simulink model "PIcomper"  (R2022b)
settings: Solver=FixedStepAuto  StartTime=0  StopTime=0.2  FixedStep=Ts  MaxStep=1e-5  RelTol=1e-5  EnableMultiTasking=on
InitFcn:
  | %% 原参数
  | Rs = 0.0135;      % 电阻
  | Ld = 5.45e-5;     % 电感
  | Ls = Ld;
  | Psi_f = 0.000639286;
  | 
  | %% 新参数
  | Rs = 0.44;
  | Ld = 0.2e-3;
  | Lq = Ld;
  | Ls = Ld;
  | Psi_f = 0.0112;
  | 
  | %% 公共参数
  | Ts = 1e-6;        % 采样时间
  | theta0 = 1.5;
  | F = 0;
  | P = 7;    % 磁极对数
  | np = P;
  | J = 1.05e-5;
  | Ud = 180; % 直流侧逆变电压。
undefined symbols (not defined in the file or in its folder): DiscIntNeverNeededParam
libraries: spsControlledVoltageSourceLib x6, spsMosfetLib x6, simulink x6, spsSeriesRLCBranchLib x3, spsCurrentMeasurementLib x3, spsVoltageMeasurementLib x3, spsDCVoltageSourceLib x1, spspowerguiLib x1, slpidlib x1, mcbcontrolslib x1
settings Model: Creator=hengst  LastModifiedBy=Administrator
settings SolverCC: AlgebraicLoopSolver=TrustRegion  AutoInsertRateTranBlk=on
settings DataIOCC: ReturnWorkspaceOutputs=off
settings OptimizationCC: LifeSpan=inf
settings DebuggingCC: UnconnectedInputMsg=warning  UnconnectedOutputMsg=warning  UnconnectedLineMsg=warning  SFUnexpectedBacktrackingDiag=warning  SFNoUnconditionalDefaultTransitionDiag=warning  ArithmeticOperatorsInVariantConditions=warning
settings ModelReferenceCC: EnableRefExpFcnMdlSchedulingChecks=on
settings SFSimCC: SimUseLocalCustomCode=off  CustomCodeUndefinedFunction=UseInterfaceOnly
settings RTWCC: RTWUseLocalCustomCode=off
settings CodeAppCC: StateflowObjectComments=on
settings GRTTargetCC: TargetLangStandard=C89/C90 (ANSI)
settings ConfigComp: CovMetricSettings=dw  CovSaveCumulativeToWorkspaceVar=on  CovSaveSingleToWorkspaceVar=on  CovExternalEMLEnable=off
settings SimscapeCC: SimscapeNormalizeSystem=off  SimscapeLogType=local

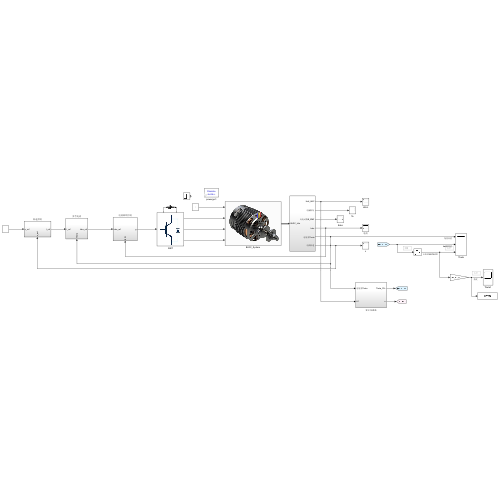
[thumbnail: Simulink's stored preview of the top-level diagram]
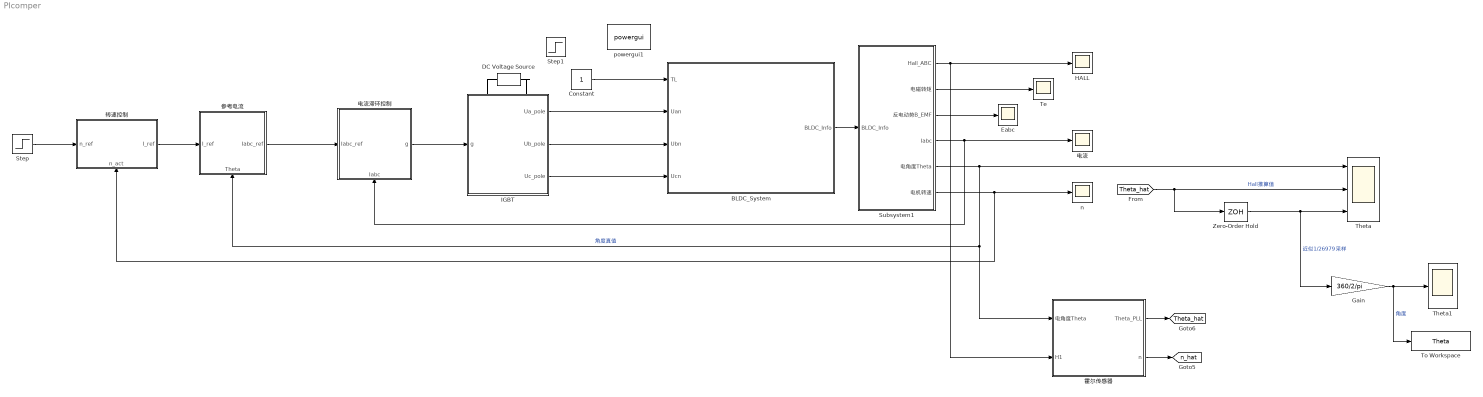
== system PIcomper ==
  BLDC_System : Subsystem
      mask Display: image('$imagefile');
  Constant : Constant
  DC Voltage Source : spsDCVoltageSourceLib/DC Voltage Source  Amplitude=Ud  Measurements=None
  Eabc : Scope
  Gain : Gain  Gain=360/2/pi
  HALL : Scope
  IGBT : Subsystem
      settings: PortSchema="{\"entries\":[{\"content\":{\"sides\":[{\"content\":{\"connectorIds\":[\"In1\"]},\"type\":\"ConnectorPlacement.EquallySpacedRectSide\",\"uuid\":\"41b52271-ff12-456f-8c0a-72ec256cd55e\"},{\"content\":{\"connectorIds\":[\"Out1\",\"Out2\",\"Out3\"],\"side\":\"RIGHT\"},\"type\":\"ConnectorPlacement.EquallySpacedRectSide\",\"uuid\":\"a3d71e7d-2158-4df1-810d-2282058bfce1\"},{\"content\":{\"connectorIds\":[\"LConn1\",\"LConn2\"],\"side\":\"TOP\"},\"type\":\"ConnectorPlacement.EquallySpacedRectSide\",\"uuid\":\"c64f7271-b3fd-4b5a-a4a2-aff74259f2ea\"}]},\"type\":\"ConnectorPlacement.EquallySpacedConnector\",\"uuid\":\"dfb04f65-d2fa-4b5c-99a8-719731ad9d2d\"}],\"packageUris\":[\"http://schema.mathworks.com/mf0/Connector/R2020b\"],\"version\":\"1.0\"}"
      mask Display: image('$imagefile'); % 使用工具条上的 "编辑图像" 进行更改。
  Step : Step  Time=0.1  Before=4000  After=2000
  Step1 : Step  Time=0.1
  Subsystem1 : Subsystem
  Te : Scope
  Theta : Scope  NumInputPorts=3
  Theta1 : Scope
  To Workspace : ToWorkspace  VariableName=Theta  SampleTime=-1
      settings: Save2DSignal=2-D array (concatenate along first dimension)
  Zero-Order Hold : ZeroOrderHold  SampleTime=3e-5
  n : Scope
  powergui1 : spspowerguiLib/powergui  Priority=1  SimulationMode=Discrete  SampleTime=Ts  frequency=60  Iterations=50  frequencyindice=0  Pbase=100e6  ErrMax=1e-4  UnitsV=kV  UnitsW=MW  buscounter=0  FunctionMessages=off  echomessages=off  EnableUseOfTLC=off  CurrentSourceSwitches=off  DisableSnubberDevices=off  DisableRonSwitches=off  DisableVfSwitches=off  DisplayEquations=off  AutomaticDiscreteSolvers=off  SolverType=Tustin/Backward Euler (TBE)  Interpol=off  ExternalGateDelay=off  methode=off  Ts=10  x0status=blocks  SPID=off  SwTol=0  HookPort=off  NonlinearTolerance=0  nMaxIteration=15  ContinueOnMaxIteration=off  RestoreLinks=warning  ResistiveCurrentMeasurement=off  Frange=[0:2:500]  Ylog=off  Xlog=on  ShowGrid=off  save=off  variable=ZData  structure=0  ZoomFFT=off  StartTime=0.0  cycles=1  DisplayStyle=1  fundamental=60  FreqAxis=off  MaxFrequency=1000  frequencyindicesteady=1  RmsSteady=1  display=off
  参考电流 : Subsystem
      settings: PortSchema="{\"entries\":[{\"content\":{\"sides\":[{\"content\":{\"connectorIds\":[\"In1\"]},\"type\":\"ConnectorPlacement.EquallySpacedRectSide\",\"uuid\":\"41f220d8-6130-485c-9e7a-1b6f64f24949\"},{\"content\":{\"connectorIds\":[\"Out1\"],\"side\":\"RIGHT\"},\"type\":\"ConnectorPlacement.EquallySpacedRectSide\",\"uuid\":\"42567a46-54e2-4998-94b6-634996524ad2\"},{\"content\":{\"side\":\"TOP\"},\"type\":\"ConnectorPlacement.EquallySpacedRectSide\",\"uuid\":\"fc447078-e630-4c42-83ce-d62d9e71be1e\"},{\"content\":{\"connectorIds\":[\"In2\"],\"side\":\"BOTTOM\"},\"type\":\"ConnectorPlacement.EquallySpacedRectSide\",\"uuid\":\"ba6e3960-44ca-42f2-94af-32e971d19e9e\"}]},\"type\":\"ConnectorPlacement.EquallySpacedConnector\",\"uuid\":\"b51f524c-61b9-4403-9c61-bea0d47ef62b\"}],\"packageUris\":[\"http://schema.mathworks.com/mf0/Connector/R2020b\"],\"version\":\"1.0\"}"
  电流 : Scope
  电流滞环控制 : Subsystem
      settings: PortSchema="{\"entries\":[{\"content\":{\"sides\":[{\"content\":{\"connectorIds\":[\"In1\"]},\"type\":\"ConnectorPlacement.EquallySpacedRectSide\",\"uuid\":\"41f220d8-6130-485c-9e7a-1b6f64f24949\"},{\"content\":{\"connectorIds\":[\"Out1\"],\"side\":\"RIGHT\"},\"type\":\"ConnectorPlacement.EquallySpacedRectSide\",\"uuid\":\"42567a46-54e2-4998-94b6-634996524ad2\"},{\"content\":{\"side\":\"TOP\"},\"type\":\"ConnectorPlacement.EquallySpacedRectSide\",\"uuid\":\"fc447078-e630-4c42-83ce-d62d9e71be1e\"},{\"content\":{\"connectorIds\":[\"In2\"],\"side\":\"BOTTOM\"},\"type\":\"ConnectorPlacement.EquallySpacedRectSide\",\"uuid\":\"84779085-48c1-4a07-a7e4-235775ba11f2\"}]},\"type\":\"ConnectorPlacement.EquallySpacedConnector\",\"uuid\":\"b51f524c-61b9-4403-9c61-bea0d47ef62b\"}],\"packageUris\":[\"http://schema.mathworks.com/mf0/Connector/R2020b\"],\"version\":\"1.0\"}"
  转速控制 : Subsystem
      settings: PortSchema="{\"entries\":[{\"content\":{\"sides\":[{\"content\":{\"connectorIds\":[\"In1\"]},\"type\":\"ConnectorPlacement.EquallySpacedRectSide\",\"uuid\":\"41f220d8-6130-485c-9e7a-1b6f64f24949\"},{\"content\":{\"connectorIds\":[\"Out1\"],\"side\":\"RIGHT\"},\"type\":\"ConnectorPlacement.EquallySpacedRectSide\",\"uuid\":\"42567a46-54e2-4998-94b6-634996524ad2\"},{\"content\":{\"side\":\"TOP\"},\"type\":\"ConnectorPlacement.EquallySpacedRectSide\",\"uuid\":\"fc447078-e630-4c42-83ce-d62d9e71be1e\"},{\"content\":{\"connectorIds\":[\"In2\"],\"side\":\"BOTTOM\"},\"type\":\"ConnectorPlacement.EquallySpacedRectSide\",\"uuid\":\"1fc4d12d-9707-4f98-a812-9cfaae9f9679\"}]},\"type\":\"ConnectorPlacement.EquallySpacedConnector\",\"uuid\":\"b51f524c-61b9-4403-9c61-bea0d47ef62b\"}],\"packageUris\":[\"http://schema.mathworks.com/mf0/Connector/R2020b\"],\"version\":\"1.0\"}"
  霍尔传感器 : Subsystem
  tag scope: Theta_hat=global, n_hat=global
  wires:
  参考电流/1(Iabc_ref) -> 电流滞环控制/1(Iabc_ref)
  电流滞环控制/1(g) -> IGBT/1(g)
  Subsystem1/6(电机转速) -> n/1, 转速控制/2(n_act)
  转速控制/1(I_ref) -> 参考电流/1(I_ref)
  Subsystem1/1(Hall_ABC) -> 霍尔传感器/2(H1), HALL/1
  BLDC_System/1(BLDC_Info) -> Subsystem1/1(BLDC_Info)
  Subsystem1/2(电磁转矩) -> Te/1
  Subsystem1/5(电角度Theta) -> Theta/1, 霍尔传感器/1(电角度Theta), 参考电流/2(Theta)  "角度真值"
  Subsystem1/4(Iabc) -> 电流/1, 电流滞环控制/2(Iabc)
  IGBT/1(Ua_pole) -> BLDC_System/2(Uan)
  IGBT/2(Ub_pole) -> BLDC_System/3(Ubn)
  IGBT/3(Uc_pole) -> BLDC_System/4(Ucn)
  Subsystem1/3(反电动势B_EMF) -> Eabc/1
  霍尔传感器/2(n) -> [n_hat]
  霍尔传感器/1(Theta_PLL) -> [Theta_hat]
  [Theta_hat] -> Zero-Order Hold/1, Theta/2  "Hall推算值"
  Zero-Order Hold/1 -> Gain/1, Theta/3  "近似1/26979采样"
  Gain/1 -> To Workspace/1, Theta1/1  "角度"
  Constant/1 -> BLDC_System/1(TL)
  Step/1 -> 转速控制/1(n_ref)
  connections:
  DC Voltage Source/RConn1 -- IGBT/LConn1
  DC Voltage Source/LConn1 -- IGBT/LConn2

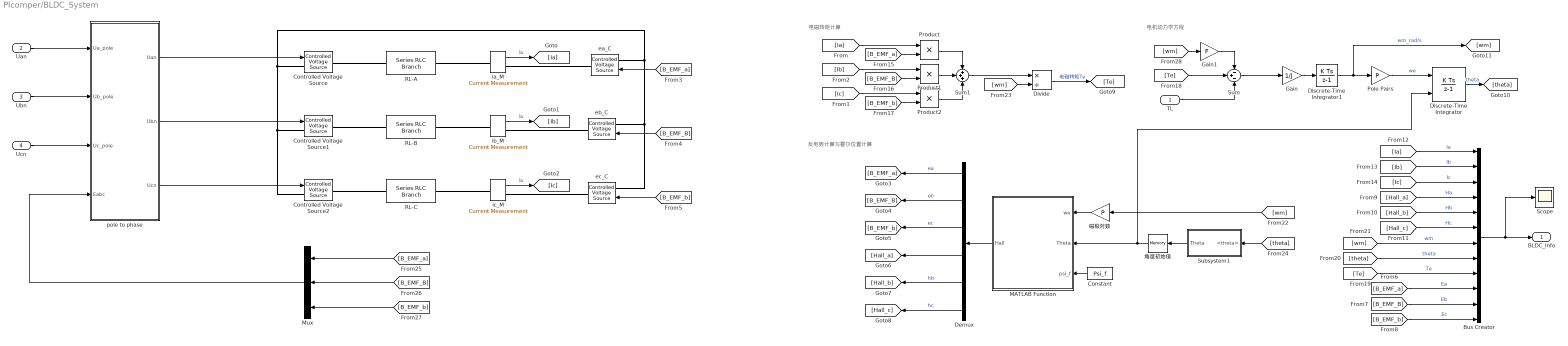
== system PIcomper/BLDC_System ==
  note: 反电势计算与霍尔位置计算
  note: 电磁转矩计算
  note: 电机动力学方程
  TL : Inport
  Uan : Inport  Port=2
  Ubn : Inport  Port=3
  Ucn : Inport  Port=4
  Bus Creator : BusCreator  Inputs=12
  Constant : Constant  Value=Psi_f
  Controlled Voltage Source : spsControlledVoltageSourceLib/Controlled Voltage Source  Initialize=on  Source_Type=AC  Amplitude=0  Phase=0  Frequency=0  Measurements=None
  Controlled Voltage Source1 : spsControlledVoltageSourceLib/Controlled Voltage Source  Initialize=on  Source_Type=AC  Amplitude=0  Phase=0  Frequency=0  Measurements=None
  Controlled Voltage Source2 : spsControlledVoltageSourceLib/Controlled Voltage Source  Initialize=on  Source_Type=AC  Amplitude=0  Phase=0  Frequency=0  Measurements=None
  Demux : Demux  Outputs=6
  Discrete-Time Integrator : DiscreteIntegrator  InitialConditionSource=external  SampleTime=-1  ICPrevOutput=DiscIntNeverNeededParam  ICPrevScaledInput=DiscIntNeverNeededParam
  Discrete-Time Integrator1 : DiscreteIntegrator  InitialCondition=1e-5  SampleTime=-1  ICPrevOutput=DiscIntNeverNeededParam  ICPrevScaledInput=DiscIntNeverNeededParam
  Divide : Product  Inputs=*/
  Gain : Gain  Gain=1/J
  Gain1 : Gain  Gain=F
  MATLAB Function : MATLAB Function  TreatAsAtomicUnit=on
  Mux : Mux  Inputs=3
  Pole Pairs : Gain  Gain=P
  Product : Product
  Product1 : Product
  Product2 : Product
  RL-A : spsSeriesRLCBranchLib/Series RLC Branch  LConnTagsString=__new0  RConnTagsString=__new0  BranchType=RL  Resistance=Rs  Inductance=Ls  SetiL0=off  InitialCurrent=0  Capacitance=1e-6  Setx0=off  InitialVoltage=0  Measurements=Branch voltage and current
  RL-B : spsSeriesRLCBranchLib/Series RLC Branch  LConnTagsString=__new0  RConnTagsString=__new0  BranchType=RL  Resistance=Rs  Inductance=Ls  SetiL0=off  InitialCurrent=0  Capacitance=1e-6  Setx0=off  InitialVoltage=0  Measurements=Branch voltage and current
  RL-C : spsSeriesRLCBranchLib/Series RLC Branch  LConnTagsString=__new0  RConnTagsString=__new0  BranchType=RL  Resistance=Rs  Inductance=Ls  SetiL0=off  InitialCurrent=0  Capacitance=1e-6  Setx0=off  InitialVoltage=0  Measurements=Branch voltage and current
  Scope : Scope
  Subsystem1 : Subsystem
  Sum : Sum  Inputs=-+-
  Sum1 : Sum  Inputs=+++
  ea_C : spsControlledVoltageSourceLib/Controlled Voltage Source  Initialize=on  Source_Type=AC  Amplitude=0  Phase=0  Frequency=0  Measurements=None
  eb_C : spsControlledVoltageSourceLib/Controlled Voltage Source  Initialize=on  Source_Type=AC  Amplitude=0  Phase=0  Frequency=0  Measurements=None
  ec_C : spsControlledVoltageSourceLib/Controlled Voltage Source  Initialize=on  Source_Type=AC  Amplitude=0  Phase=0  Frequency=0  Measurements=None
  ia_M : spsCurrentMeasurementLib/Current Measurement  PhasorSimulation=off  OutputType=Complex  PSBequivalent=0
  ib_M : spsCurrentMeasurementLib/Current Measurement  PhasorSimulation=off  OutputType=Complex  PSBequivalent=0
  ic_M : spsCurrentMeasurementLib/Current Measurement  PhasorSimulation=off  OutputType=Complex  PSBequivalent=0
  pole to phase : Subsystem
  磁极对数 : Gain  Gain=P
  角度初始值 : Memory  InitialCondition=theta0  InheritSampleTime=on
  BLDC_Info : Outport  VectorParamsAs1DForOutWhenUnconnected=off
  wires:
  ia_M/1 -> [Ia]  "ia"
  Product1/1 -> Sum1/2
  Product/1 -> Sum1/1
  Product2/1 -> Sum1/3
  Sum1/1 -> Divide/1
  Sum/1 -> Gain/1
  Discrete-Time Integrator1/1 -> [wm], Pole Pairs/1  "wm_rad/s"
  Pole Pairs/1 -> Discrete-Time Integrator/1  "we"
  MATLAB Function/1(Hall) -> Demux/1
  Gain/1 -> Discrete-Time Integrator1/1
  Subsystem1/1(Theta) -> 角度初始值/1
  [Ia] -> Product/1
  ib_M/1 -> [Ib]  "ia"
  ic_M/1 -> [Ic]  "ia"
  [Ib] -> Product1/1
  [Ic] -> Product2/1
  Demux/1 -> [B_EMF_a]  "ea"
  Demux/2 -> [B_EMF_B]  "eb"
  Demux/3 -> [B_EMF_b]  "ec"
  [B_EMF_a] -> Bus Creator/10  "Ea"
  [B_EMF_B] -> Bus Creator/11  "Eb"
  [B_EMF_b] -> Bus Creator/12  "Ec"
  [B_EMF_a] -> ea_C/1
  [B_EMF_B] -> eb_C/1
  [B_EMF_b] -> ec_C/1
  Demux/4 -> [Hall_a]
  Demux/5 -> [Hall_b]  "hb"
  Demux/6 -> [Hall_c]  "hc"
  [Hall_a] -> Bus Creator/4  "Ha"
  [Hall_b] -> Bus Creator/5  "Hb"
  [Hall_c] -> Bus Creator/6  "Hc"
  [Ia] -> Bus Creator/1  "Ia"
  [Ib] -> Bus Creator/2  "Ib"
  [Ic] -> Bus Creator/3  "Ic"
  [B_EMF_a] -> Product/2
  [B_EMF_B] -> Product1/2
  [B_EMF_b] -> Product2/2
  Divide/1 -> [Te]  "电磁转矩Te"
  [Te] -> Bus Creator/9  "Te"
  Discrete-Time Integrator/1 -> [theta]  "theta"
  [theta] -> Bus Creator/8  "theta"
  [wm] -> Bus Creator/7  "wm"
  [wm] -> Divide/2
  [wm] -> 磁极对数/1
  [theta] -> Subsystem1/1(<theta>)
  磁极对数/1 -> MATLAB Function/1(we)
  Constant/1 -> MATLAB Function/3(psi_f)
  Bus Creator/1 -> Scope/1, BLDC_Info/1
  Mux/1 -> pole to phase/4(Eabc)
  Ubn/1 -> pole to phase/2(Ub_pole)
  pole to phase/2(Ubn) -> Controlled Voltage Source1/1
  Uan/1 -> pole to phase/1(Ua_pole)
  Ucn/1 -> pole to phase/3("Uc_pole ")
  pole to phase/1(Uan) -> Controlled Voltage Source/1
  pole to phase/3(Ucn) -> Controlled Voltage Source2/1
  [B_EMF_a] -> Mux/1
  [B_EMF_B] -> Mux/2
  [B_EMF_b] -> Mux/3
  [Te] -> Sum/2
  TL/1 -> Sum/3
  [wm] -> Gain1/1
  Gain1/1 -> Sum/1
  角度初始值/1 -> Discrete-Time Integrator/2, MATLAB Function/2(Theta)
  connections:
  Controlled Voltage Source/RConn1 -- RL-A/LConn1
  RL-B/LConn1 -- Controlled Voltage Source1/RConn1
  RL-C/LConn1 -- Controlled Voltage Source2/RConn1
  RL-A/RConn1 -- ia_M/LConn1
  ic_M/LConn1 -- RL-C/RConn1
  ia_M/RConn1 -- ea_C/RConn1
  ea_C/LConn1 -- Controlled Voltage Source/LConn1 -- Controlled Voltage Source2/LConn1 -- Controlled Voltage Source1/LConn1 -- ec_C/LConn1 -- eb_C/LConn1
  RL-B/RConn1 -- ib_M/LConn1
  ib_M/RConn1 -- eb_C/RConn1
  ic_M/RConn1 -- ec_C/RConn1

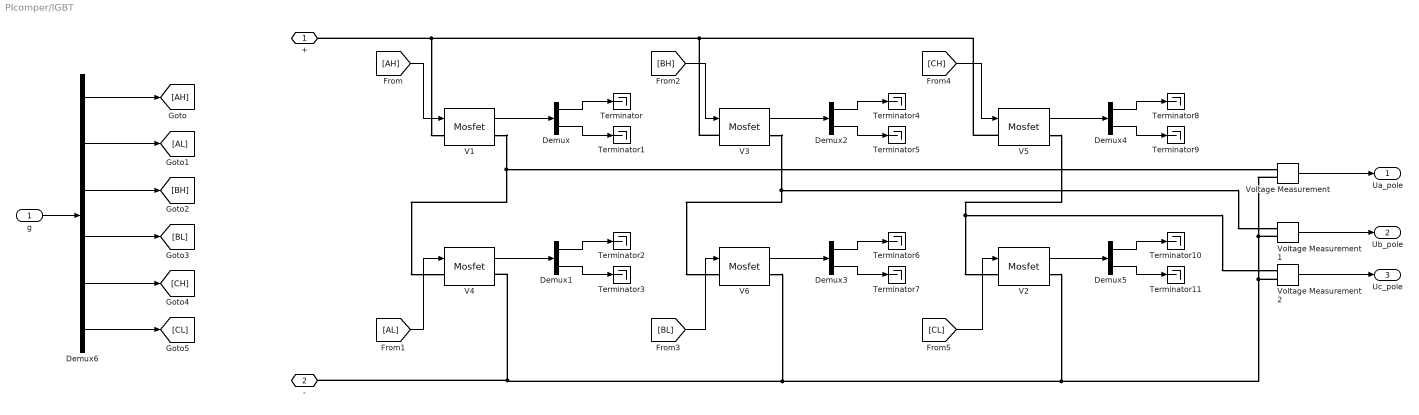
== system PIcomper/IGBT ==
  g : Inport
  Demux{,1..5} (6 alike) : Demux  Outputs=2
  Demux6 : Demux  Outputs=6
  Terminator{,1..11} (12 alike) : Terminator
  V{1..6} (6 alike) : spsMosfetLib/Mosfet  Ron=1e-3  Lon=0  Rd=0.01  Vfd=0  IC=0  Rs=5000  Cs=1e-6  Measurements=on
  Voltage Measurement : spsVoltageMeasurementLib/Voltage Measurement  PhasorSimulation=off  OutputType=Complex  PSBequivalent=0
  Voltage Measurement1 : spsVoltageMeasurementLib/Voltage Measurement  PhasorSimulation=off  OutputType=Complex  PSBequivalent=0
  Voltage Measurement2 : spsVoltageMeasurementLib/Voltage Measurement  PhasorSimulation=off  OutputType=Complex  PSBequivalent=0
  + : PMIOPort  Side=Left
  - : PMIOPort  Port=2  Side=Left
  Ua_pole : Outport  VectorParamsAs1DForOutWhenUnconnected=off
  Ub_pole : Outport  Port=2  VectorParamsAs1DForOutWhenUnconnected=off
  Uc_pole : Outport  Port=3  VectorParamsAs1DForOutWhenUnconnected=off
  wires:
  V5/1 -> Demux4/1
  Demux4/1 -> Terminator8/1
  Demux4/2 -> Terminator9/1
  V2/1 -> Demux5/1
  Demux5/1 -> Terminator10/1
  Demux5/2 -> Terminator11/1
  Demux1/2 -> Terminator3/1
  Demux1/1 -> Terminator2/1
  V4/1 -> Demux1/1
  V3/1 -> Demux2/1
  Demux2/1 -> Terminator4/1
  Demux2/2 -> Terminator5/1
  V6/1 -> Demux3/1
  Demux3/1 -> Terminator6/1
  Demux3/2 -> Terminator7/1
  Demux/2 -> Terminator1/1
  V1/1 -> Demux/1
  Demux/1 -> Terminator/1
  [BH] -> V3/1
  [BL] -> V6/1
  [AL] -> V4/1
  [AH] -> V1/1
  [CL] -> V2/1
  [CH] -> V5/1
  g/1 -> Demux6/1
  Demux6/1 -> [AH]
  Demux6/2 -> [AL]
  Demux6/3 -> [BH]
  Demux6/4 -> [BL]
  Demux6/5 -> [CH]
  Demux6/6 -> [CL]
  Voltage Measurement/1 -> Ua_pole/1
  Voltage Measurement1/1 -> Ub_pole/1
  Voltage Measurement2/1 -> Uc_pole/1
  connections:
  V5/RConn1 -- Voltage Measurement2/LConn1 -- V2/LConn1
  V1/RConn1 -- Voltage Measurement/LConn1 -- V4/LConn1
  V3/RConn1 -- Voltage Measurement1/LConn1 -- V6/LConn1
  Voltage Measurement2/LConn2 -- Voltage Measurement1/LConn2 -- Voltage Measurement/LConn2 -- V2/RConn1 -- V6/RConn1 -- -/RConn1 -- V4/RConn1
  V5/LConn1 -- V3/LConn1 -- +/RConn1 -- V1/LConn1

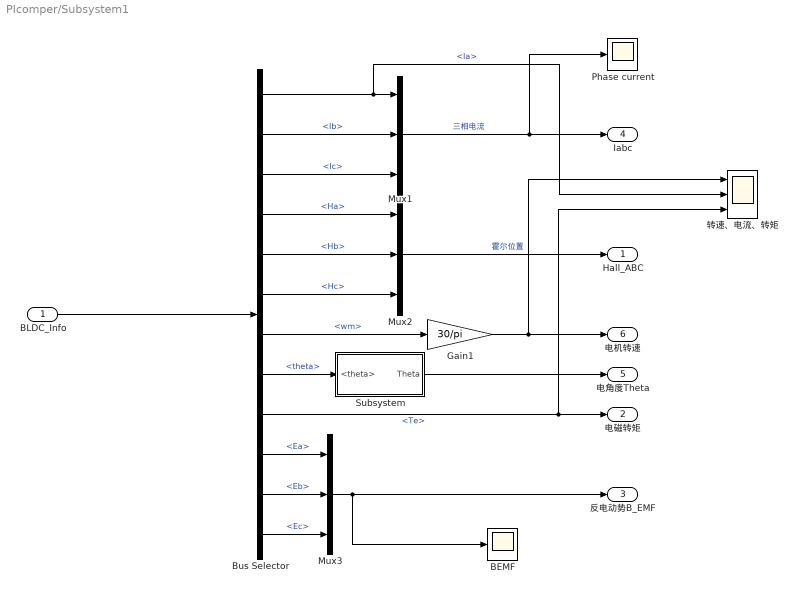
== system PIcomper/Subsystem1 ==
  BLDC_Info : Inport
  BEMF : Scope
  Bus Selector : BusSelector  OutputSignals=Ia,Ib,Ic,Ha,Hb,Hc,wm,theta,Te,Ea,Eb,Ec
  Gain1 : Gain  Gain=30/pi
  Mux1 : Mux  Inputs=3
  Mux2 : Mux  Inputs=3
  Mux3 : Mux  Inputs=3
  Phase current : Scope
  Subsystem : Subsystem
  转速、电流、转矩 : Scope  NumInputPorts=3
  Hall_ABC : Outport  VectorParamsAs1DForOutWhenUnconnected=off
  电磁转矩 : Outport  Port=2  VectorParamsAs1DForOutWhenUnconnected=off
  反电动势B_EMF : Outport  Port=3  VectorParamsAs1DForOutWhenUnconnected=off
  Iabc : Outport  Port=4  VectorParamsAs1DForOutWhenUnconnected=off
  电角度Theta : Outport  Port=5  VectorParamsAs1DForOutWhenUnconnected=off
  电机转速 : Outport  Port=6  VectorParamsAs1DForOutWhenUnconnected=off
  wires:
  Bus Selector/4 -> Mux2/1  "<Ha>"
  Bus Selector/10 -> Mux3/1  "<Ea>"
  Bus Selector/2 -> Mux1/2  "<Ib>"
  Mux3/1 -> 反电动势B_EMF/1, BEMF/1
  Bus Selector/11 -> Mux3/2  "<Eb>"
  Mux1/1 -> Iabc/1, Phase current/1  "三相电流"
  Gain1/1 -> 转速、电流、转矩/1, 电机转速/1
  Bus Selector/8 -> Subsystem/1(<theta>)  "<theta>"
  Bus Selector/9 -> 转速、电流、转矩/3, 电磁转矩/1  "<Te>"
  Bus Selector/6 -> Mux2/3  "<Hc>"
  Bus Selector/12 -> Mux3/3  "<Ec>"
  Bus Selector/7 -> Gain1/1  "<wm>"
  Subsystem/1(Theta) -> 电角度Theta/1
  Mux2/1 -> Hall_ABC/1  "霍尔位置"
  BLDC_Info/1 -> Bus Selector/1
  Bus Selector/5 -> Mux2/2  "<Hb>"
  Bus Selector/3 -> Mux1/3  "<Ic>"
  Bus Selector/1 -> 转速、电流、转矩/2, Mux1/1  "<Ia>"

== system PIcomper/参考电流 ==
  I_ref : Inport
  Theta : Inport  Port=2
  当前位置+参考电流生成三相参考电流 : MATLAB Function  TreatAsAtomicUnit=on
  Iabc_ref : Outport  VectorParamsAs1DForOutWhenUnconnected=off
  wires:
  I_ref/1 -> 当前位置+参考电流生成三相参考电流/1(I_ref)
  Theta/1 -> 当前位置+参考电流生成三相参考电流/2(theta)
  当前位置+参考电流生成三相参考电流/1(Iabc_Ref) -> Iabc_ref/1

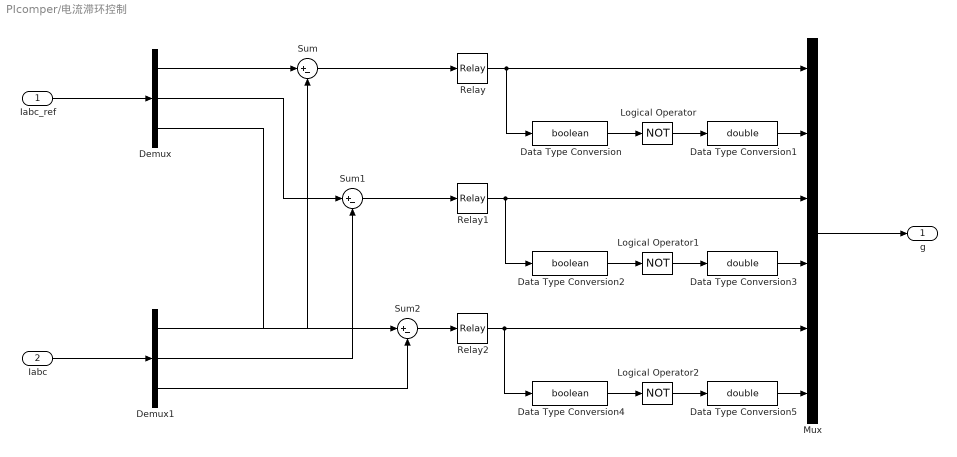
== system PIcomper/电流滞环控制 ==
  Iabc_ref : Inport
  Iabc : Inport  Port=2
  Data Type Conversion : DataTypeConversion  OutDataTypeStr=boolean  SaturateOnIntegerOverflow=off  RndMeth=Floor
  Data Type Conversion1 : DataTypeConversion  OutDataTypeStr=double  SaturateOnIntegerOverflow=off  RndMeth=Floor
  Data Type Conversion2 : DataTypeConversion  OutDataTypeStr=boolean  SaturateOnIntegerOverflow=off  RndMeth=Floor
  Data Type Conversion3 : DataTypeConversion  OutDataTypeStr=double  SaturateOnIntegerOverflow=off  RndMeth=Floor
  Data Type Conversion4 : DataTypeConversion  OutDataTypeStr=boolean  SaturateOnIntegerOverflow=off  RndMeth=Floor
  Data Type Conversion5 : DataTypeConversion  OutDataTypeStr=double  SaturateOnIntegerOverflow=off  RndMeth=Floor
  Demux : Demux  Outputs=3
  Demux1 : Demux  Outputs=3
  Logical Operator : Logic  Operator=NOT  AllPortsSameDT=off  OutDataTypeStr=boolean
  Logical Operator1 : Logic  Operator=NOT  AllPortsSameDT=off  OutDataTypeStr=boolean
  Logical Operator2 : Logic  Operator=NOT  AllPortsSameDT=off  OutDataTypeStr=boolean
  Mux : Mux  Inputs=6
  Relay : Relay  OnSwitchValue=0.005  OffSwitchValue=-0.005
  Relay1 : Relay  OnSwitchValue=0.005  OffSwitchValue=-0.005
  Relay2 : Relay  OnSwitchValue=0.005  OffSwitchValue=-0.005
  Sum : Sum  Inputs=|+-
  Sum1 : Sum  Inputs=|+-
  Sum2 : Sum  Inputs=|+-
  g : Outport  VectorParamsAs1DForOutWhenUnconnected=off
  wires:
  Relay/1 -> Mux/1, Data Type Conversion/1
  Logical Operator/1 -> Data Type Conversion1/1
  Data Type Conversion5/1 -> Mux/6
  Data Type Conversion/1 -> Logical Operator/1
  Data Type Conversion3/1 -> Mux/4
  Data Type Conversion1/1 -> Mux/2
  Relay1/1 -> Mux/3, Data Type Conversion2/1
  Mux/1 -> g/1
  Relay2/1 -> Data Type Conversion4/1, Mux/5
  Sum/1 -> Relay/1
  Data Type Conversion2/1 -> Logical Operator1/1
  Logical Operator1/1 -> Data Type Conversion3/1
  Data Type Conversion4/1 -> Logical Operator2/1
  Logical Operator2/1 -> Data Type Conversion5/1
  Sum1/1 -> Relay1/1
  Sum2/1 -> Relay2/1
  Demux/1 -> Sum/1
  Iabc_ref/1 -> Demux/1
  Demux/2 -> Sum1/1
  Demux/3 -> Sum2/1
  Iabc/1 -> Demux1/1
  Demux1/1 -> Sum/2
  Demux1/2 -> Sum1/2
  Demux1/3 -> Sum2/2

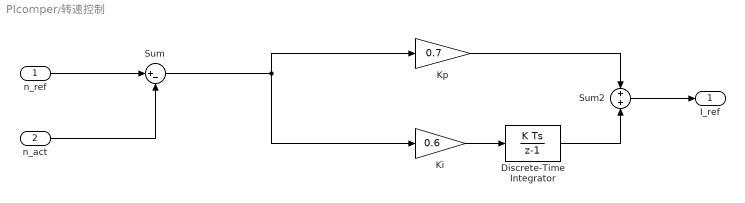
== system PIcomper/转速控制 ==
  n_ref : Inport
  n_act : Inport  Port=2
  Discrete-Time Integrator : DiscreteIntegrator  SampleTime=-1  LimitOutput=on  UpperSaturationLimit=55  LowerSaturationLimit=-55  ICPrevOutput=DiscIntNeverNeededParam  ICPrevScaledInput=DiscIntNeverNeededParam
  Ki : Gain  Gain=0.6
  Kp : Gain  Gain=0.7
  Sum : Sum  Inputs=|+-
  Sum2 : Sum
  I_ref : Outport  VectorParamsAs1DForOutWhenUnconnected=off
  wires:
  n_act/1 -> Sum/2
  n_ref/1 -> Sum/1
  Discrete-Time Integrator/1 -> Sum2/2
  Kp/1 -> Sum2/1
  Sum2/1 -> I_ref/1
  Sum/1 -> Ki/1, Kp/1
  Ki/1 -> Discrete-Time Integrator/1

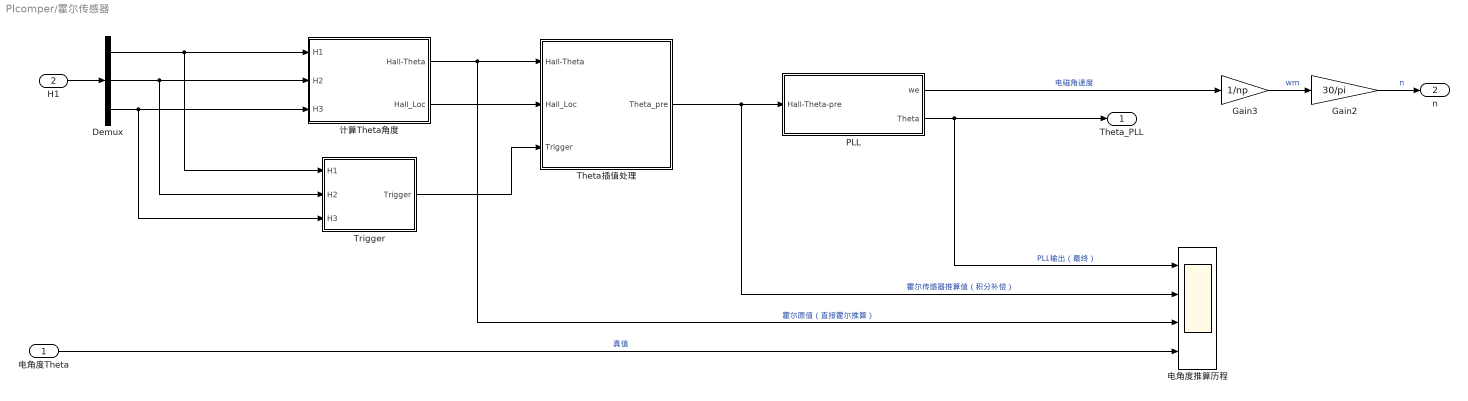
== system PIcomper/霍尔传感器 ==
  电角度Theta : Inport
  H1 : Inport  Port=2
  Demux : Demux  Outputs=3
  Gain2 : Gain  Gain=30/pi
  Gain3 : Gain  Gain=1/np
  PLL : Subsystem
  Theta插值处理 : Subsystem
  Trigger : Subsystem
  电角度推算历程 : Scope  NumInputPorts=4
  计算Theta角度 : Subsystem
  Theta_PLL : Outport
  n : Outport  Port=2
  wires:
  Demux/3 -> Trigger/3(H3), 计算Theta角度/3(H3)
  Demux/2 -> Trigger/2(H2), 计算Theta角度/2(H2)
  Trigger/1(Trigger) -> Theta插值处理/3(Trigger)
  计算Theta角度/1(Hall-Theta) -> 电角度推算历程/3, Theta插值处理/1(Hall-Theta)  "霍尔原值（直接霍尔推算）"
  Gain3/1 -> Gain2/1  "wm"
  Gain2/1 -> n/1  "n"
  PLL/1(we) -> Gain3/1  "电磁角速度"
  PLL/2(Theta) -> 电角度推算历程/1, Theta_PLL/1  "PLL输出（最终）"
  Theta插值处理/1(Theta_pre) -> PLL/1(Hall-Theta-pre), 电角度推算历程/2  "霍尔传感器推算值（积分补偿）"
  Demux/1 -> Trigger/1(H1), 计算Theta角度/1(H1)
  H1/1 -> Demux/1
  计算Theta角度/2(Hall_Loc) -> Theta插值处理/2(Hall_Loc)
  电角度Theta/1 -> 电角度推算历程/4  "真值"

== system PIcomper/BLDC_System/Subsystem1 ==
  <theta> : Inport
  Constant1 : Constant  Value=2*pi
  Math Function : Math  Operator=rem  SignedPower=on
  Theta : Outport
  wires:
  Constant1/1 -> Math Function/2
  <theta>/1 -> Math Function/1
  Math Function/1 -> Theta/1

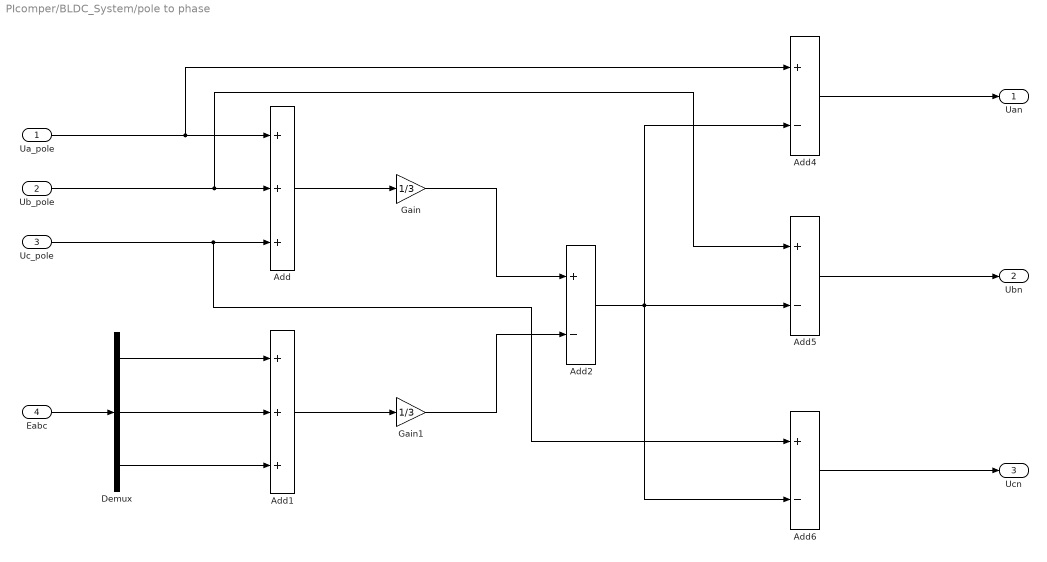
== system PIcomper/BLDC_System/pole to phase ==
  Ua_pole : Inport
  Ub_pole : Inport  Port=2
  "Uc_pole " : Inport  Port=3
  Eabc : Inport  Port=4
  Add : Sum  Inputs=3
  Add1 : Sum  Inputs=3
  Add{2,4..6} (4 alike) : Sum  Inputs=+-
  Demux : Demux  Outputs=3
  Gain : Gain  Gain=1/3
  Gain1 : Gain  Gain=1/3
  Uan : Outport  VectorParamsAs1DForOutWhenUnconnected=off
  Ubn : Outport  Port=2  VectorParamsAs1DForOutWhenUnconnected=off
  Ucn : Outport  Port=3  VectorParamsAs1DForOutWhenUnconnected=off
  wires:
  "Uc_pole "/1 -> Add6/1, Add/3
  Gain/1 -> Add2/1
  Add1/1 -> Gain1/1
  Add6/1 -> Ucn/1
  Ua_pole/1 -> Add4/1, Add/1
  Ub_pole/1 -> Add5/1, Add/2
  Add/1 -> Gain/1
  Demux/1 -> Add1/1
  Demux/3 -> Add1/3
  Demux/2 -> Add1/2
  Add2/1 -> Add6/2, Add5/2, Add4/2
  Add4/1 -> Uan/1
  Add5/1 -> Ubn/1
  Gain1/1 -> Add2/2
  Eabc/1 -> Demux/1

== system PIcomper/Subsystem1/Subsystem ==
  <theta> : Inport
  Constant1 : Constant  Value=2*pi
  Math Function : Math  Operator=rem  SignedPower=on
  Theta : Outport
  wires:
  Constant1/1 -> Math Function/2
  <theta>/1 -> Math Function/1
  Math Function/1 -> Theta/1

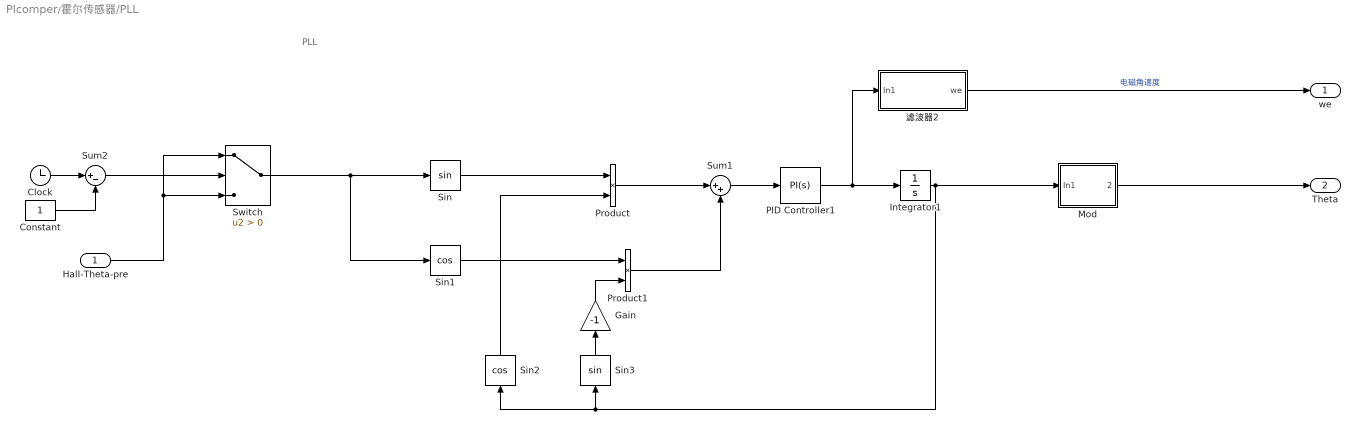
== system PIcomper/霍尔传感器/PLL ==
  note: PLL
  Hall-Theta-pre : Inport
  Clock : Clock
  Constant : Constant
  Gain : Gain  Gain=-1
  Integrator1 : Integrator
  Mod : Subsystem
  PID Controller1 : slpidlib/PID Controller  Controller=PI  Form=Parallel  TimeDomain=Continuous-time  UseExternalTs=off  SampleTime=-1  IntegratorMethod=Forward Euler  FilterMethod=Forward Euler  ControllerParametersSource=internal  P=50000  I=50000  UseKiTs=off  D=0  N=100  UseFilter=on  TunerSelectOption=Transfer Function Based (PID Tuner App)  InitialConditionSource=internal  InitialConditionForIntegrator=0  InitialConditionForFilter=0  DifferentiatorICPrevScaledInput=0  ExternalReset=none  TrackingMode=off  Kt=1  LimitOutput=off  SatLimitsSource=internal  UpperSaturationLimit=inf  LowerSaturationLimit=-inf  LinearizeAsGain=on  AntiWindupMode=none  Kb=1  LimitIntegrator=off  UpperIntegratorSaturationLimit=inf  LowerIntegratorSaturationLimit=-inf  POutMin=[]  POutMax=[]  IOutMin=[]  IOutMax=[]  DOutMin=[]  DOutMax=[]  NOutMin=[]  NOutMax=[]  SumOutMin=[]  SumOutMax=[]  SaturationOutMin=[]  SaturationOutMax=[]  PParamMin=[]  PParamMax=[]  IParamMin=[]  IParamMax=[]  DParamMin=[]  DParamMax=[]  NParamMin=[]  NParamMax=[]  KbParamMin=[]  KbParamMax=[]  KtParamMin=[]  KtParamMax=[]  KbOutMin=[]  KbOutMax=[]  KtOutMin=[]  KtOutMax=[]  IntegratorOutMin=[]  IntegratorOutMax=[]  FilterOutMin=[]  FilterOutMax=[]  SumI1OutMin=[]  SumI1OutMax=[]  SumI2OutMin=[]  SumI2OutMax=[]  SumI3OutMin=[]  SumI3OutMax=[]  SumI4OutMin=[]  SumI4OutMax=[]  SumDOutMin=[]  SumDOutMax=[]  DifferentiatorOutMin=[]  DifferentiatorOutMax=[]  FilterDiffOutCoefMin=[]  FilterDiffOutCoefMax=[]  ReciprocalOutMin=[]  ReciprocalOutMax=[]  SumDenOutMin=[]  SumDenOutMax=[]  SumNumOutMin=[]  SumNumOutMax=[]  DivideOutMin=[]  DivideOutMax=[]  UdiffTsProdOutMin=[]  UdiffTsProdOutMax=[]  NTsProdOutMin=[]  NTsProdOutMax=[]  UintegralTsProdOutMin=[]  UintegralTsProdOutMax=[]  UngainTsProdOutMin=[]  UngainTsProdOutMax=[]  ClampingZeroOutDataTypeStr=Inherit: Inherit via back propagation  ClampingZeroOutMin=[]  ClampingZeroOutMax=[]  FilterDenConstantOutDataTypeStr=Inherit: Inherit via back propagation  FilterDenConstantOutMin=[]  FilterDenConstantOutMax=[]  PCopyOutDataTypeStr=Inherit: Inherit via back propagation  PCopyOutMin=[]  PCopyOutMax=[]  NCopyOutDataTypeStr=Inherit: Inherit via back propagation  NCopyOutMin=[]  NCopyOutMax=[]  IntegratorContinuousStateAttributes=''  IntegratorStateMustResolveToSignalObject=off  IntegratorRTWStateStorageClass=Auto  FilterContinuousStateAttributes=''  FilterStateMustResolveToSignalObject=off  FilterRTWStateStorageClass=Auto  ParallelPVariant=InternalParameters  IdealPVariant=Disabled  IVariant=InternalParameters  DVariant=Disabled  IntegratorVariant=Continuous  SatVariant=Disabled  AWVariant=Passthrough  PCopyVariant=Disabled  TRVariant=Disabled  FdbkBlocksVariant=Forward  IdealPFdbkVariant=Disabled  SatFdbkVariant=Disabled  DerivativeFilterVariant=Disabled  NVariant=Disabled  NCopyVariant=Disabled_SignalSpec  FilterICVariant=Disabled  IntegratorICVariant=InternalICs  ExternalResetVariant=Disabled  TRSumVariant=Passthrough  SumFdbkVariant=Disabled  SumVariant=Sum_PI  TsampFilterVariant=InternalTs  TsampNgainVariant=Passthrough  TsampIntegralVariant=Passthrough  ExternalSaturationOutDataTypeStr=Inherit: Same as second input
  Product : Product
  Product1 : Product
  Sin : Trigonometry
  Sin1 : Trigonometry  Operator=cos
  Sin2 : Trigonometry  Operator=cos
  Sin3 : Trigonometry
  Sum1 : Sum  Inputs=|++
  Sum2 : Sum  Inputs=|+-
  Switch : Switch  Criteria=u2 > Threshold  SaturateOnIntegerOverflow=off  InputSameDT=off
  滤波器2 : Subsystem
  we : Outport
  Theta : Outport  Port=2
  wires:
  Hall-Theta-pre/1 -> Switch/3, Switch/1
  Sin/1 -> Product/1
  Sin2/1 -> Product/2
  Sin1/1 -> Product1/1
  Sin3/1 -> Gain/1
  Gain/1 -> Product1/2
  Product/1 -> Sum1/1
  Product1/1 -> Sum1/2
  Sum1/1 -> PID Controller1/1
  PID Controller1/1 -> 滤波器2/1(In1), Integrator1/1
  Integrator1/1 -> Sin2/1, Sin3/1, Mod/1(In1)
  滤波器2/1(we) -> we/1  "电磁角速度"
  Clock/1 -> Sum2/1
  Sum2/1 -> Switch/2
  Constant/1 -> Sum2/2
  Switch/1 -> Sin1/1, Sin/1
  Mod/1(2) -> Theta/1

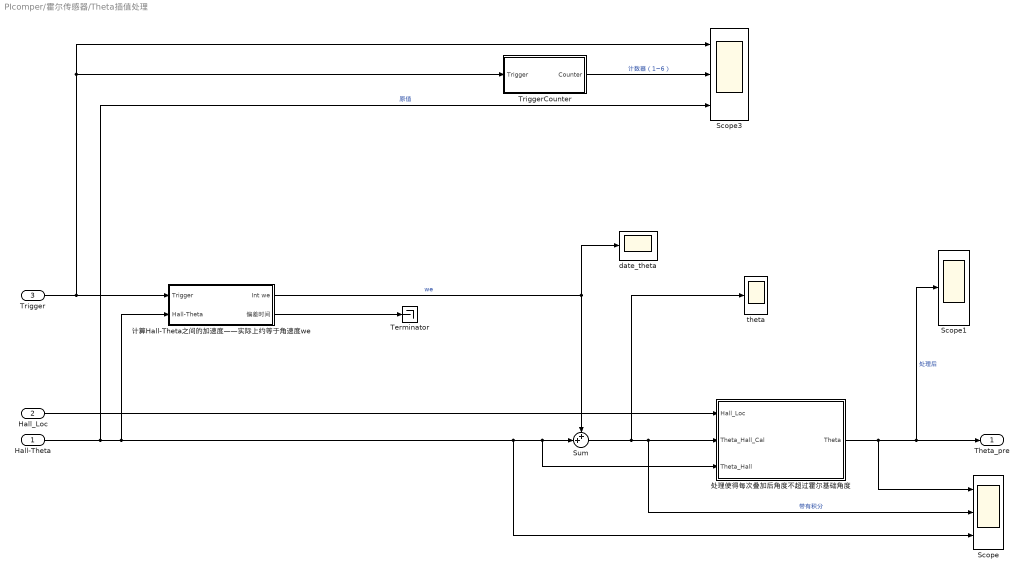
== system PIcomper/霍尔传感器/Theta插值处理 ==
  Hall-Theta : Inport
  Hall_Loc : Inport  Port=2
  Trigger : Inport  Port=3
  Scope : Scope  NumInputPorts=3
  Scope1 : Scope
  Scope3 : Scope  NumInputPorts=3
  Sum : Sum  Inputs=++|
  Terminator : Terminator
  TriggerCounter : MATLAB Function  TreatAsAtomicUnit=on
  date_theta : Scope
  theta : Scope
  处理使得每次叠加后角度不超过霍尔基础角度 : MATLAB Function  TreatAsAtomicUnit=on
  计算Hall-Theta之间的加速度——实际上约等于角速度we : Subsystem
  Theta_pre : Outport
  wires:
  计算Hall-Theta之间的加速度——实际上约等于角速度we/1(Int we) -> Sum/1, date_theta/1  "we"
  Trigger/1 -> TriggerCounter/1(Trigger), Scope3/1, 计算Hall-Theta之间的加速度——实际上约等于角速度we/1(Trigger)
  处理使得每次叠加后角度不超过霍尔基础角度/1(Theta) -> Scope/1, Scope1/1, Theta_pre/1  "处理后"
  TriggerCounter/1(Counter) -> Scope3/2  "计数器（1~6）"
  Sum/1 -> theta/1, Scope/2, 处理使得每次叠加后角度不超过霍尔基础角度/2(Theta_Hall_Cal)  "带有积分"
  Hall-Theta/1 -> Scope3/3, Scope/3, 处理使得每次叠加后角度不超过霍尔基础角度/3(Theta_Hall), Sum/2, 计算Hall-Theta之间的加速度——实际上约等于角速度we/2(Hall-Theta)  "原值"
  计算Hall-Theta之间的加速度——实际上约等于角速度we/2(偏差时间) -> Terminator/1
  Hall_Loc/1 -> 处理使得每次叠加后角度不超过霍尔基础角度/1(Hall_Loc)

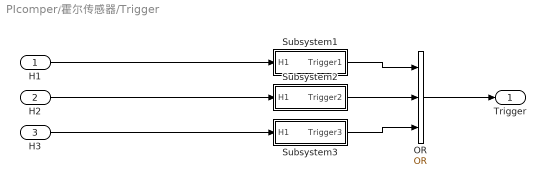
== system PIcomper/霍尔传感器/Trigger ==
  H1 : Inport
  H2 : Inport  Port=2
  H3 : Inport  Port=3
  OR : Logic  Operator=OR  Inputs=3  IconShape=distinctive  AllPortsSameDT=off  OutDataTypeStr=boolean
  Subsystem1 : Subsystem
  Subsystem2 : Subsystem
  Subsystem3 : Subsystem
  Trigger : Outport
  wires:
  H2/1 -> Subsystem2/1(H1)
  H1/1 -> Subsystem1/1(H1)
  OR/1 -> Trigger/1
  H3/1 -> Subsystem3/1(H1)
  Subsystem2/1(Trigger2) -> OR/2
  Subsystem1/1(Trigger1) -> OR/1
  Subsystem3/1(Trigger3) -> OR/3

== system PIcomper/霍尔传感器/计算Theta角度 ==
  H1 : Inport
  H2 : Inport  Port=2
  H3 : Inport  Port=3
  MATLAB Function : MATLAB Function  TreatAsAtomicUnit=on
  Mux : Mux  Inputs=3
  Hall-Theta : Outport
  Hall_Loc : Outport  Port=2
  wires:
  H2/1 -> Mux/2
  H3/1 -> Mux/3
  Mux/1 -> MATLAB Function/1(Hall_abc)
  MATLAB Function/1(theta_Hall) -> Hall-Theta/1
  H1/1 -> Mux/1
  MATLAB Function/2(theta_loc) -> Hall_Loc/1

== system PIcomper/霍尔传感器/PLL/Mod ==
  In1 : Inport
  Constant7 : Constant  Value=2*pi
  Mod : Math  Operator=mod
  2 : Outport
  wires:
  Constant7/1 -> Mod/2
  Mod/1 -> 2/1  "真值"
  In1/1 -> Mod/1

== system PIcomper/霍尔传感器/PLL/滤波器2 ==
  note: wc/(1+wc) wc增大会增大动态响应速度，但是过大会导致滤波效果不好，需要权衡
  note: 【注】滤波器会延时，导致转速延迟，不是特别建议补偿
  In1 : Inport
  Filter1 : TransferFcn  Numerator=[2000]  Denominator=[1 2000]
  Filter3 : TransferFcn  Numerator=[50]  Denominator=[1 50]
  Filter4 : TransferFcn  Numerator=[2000]  Denominator=[1 2000]
  IIR Filter : mcbcontrolslib/IIR Filter  VariantControl=Low Pass Filter  VariantSelect=Low-pass  Filter_constant=0.0001  advancedSettings=on  Ts=1e-5  cutOff_freq=1.5917
  滤波器参数对比 : Scope  NumInputPorts=4
  we : Outport
  wires:
  In1/1 -> IIR Filter/1, 滤波器参数对比/3, Filter3/1, Filter4/1
  Filter4/1 -> Filter1/1
  Filter3/1 -> 滤波器参数对比/2
  IIR Filter/1 -> we/1, 滤波器参数对比/4
  Filter1/1 -> 滤波器参数对比/1

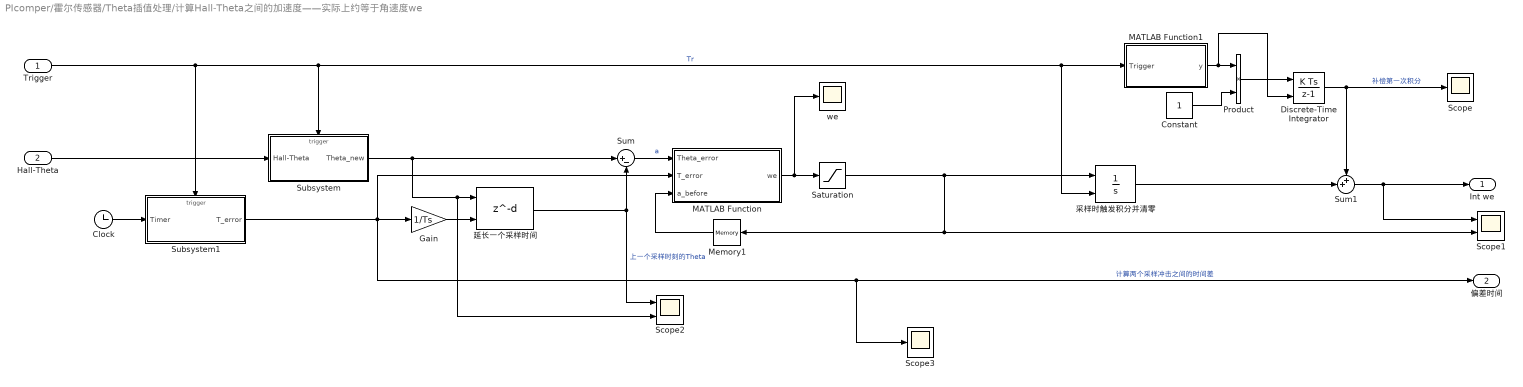
== system PIcomper/霍尔传感器/Theta插值处理/计算Hall-Theta之间的加速度——实际上约等于角速度we ==
  Trigger : Inport
  Hall-Theta : Inport  Port=2
  Clock : Clock
  Constant : Constant
  Discrete-Time Integrator : DiscreteIntegrator  ExternalReset=falling  SampleTime=-1  ICPrevOutput=DiscIntNeverNeededParam  ICPrevScaledInput=DiscIntNeverNeededParam
  Gain : Gain  Gain=1/Ts
  MATLAB Function : MATLAB Function  TreatAsAtomicUnit=on
  MATLAB Function1 : MATLAB Function  TreatAsAtomicUnit=on
  Memory1 : Memory  InitialCondition=50
  Product : Product
  Saturation : Saturate  UpperLimit=1/Ts  LowerLimit=-1/Ts
  Scope : Scope
  Scope1 : Scope  NumInputPorts=2
  Scope2 : Scope  NumInputPorts=2
  Scope3 : Scope
  Subsystem : Subsystem
  Subsystem1 : Subsystem
  Sum : Sum  Inputs=|+-
  Sum1 : Sum  Inputs=++|
  we : Scope
  延长一个采样时间 : Delay  DelayLengthSource=Input port  DelayLengthUpperLimit=100000  PreventDirectFeedthrough=on  UseCircularBuffer=on
      settings: InputPortMap=u0,p1
  采样时触发积分并清零 : Integrator  ExternalReset=rising
  Int we : Outport
  偏差时间 : Outport  Port=2
  wires:
  Hall-Theta/1 -> Subsystem/1(Hall-Theta)
  Subsystem/1(Theta_new) -> Sum/1, Scope2/2, 延长一个采样时间/1
  Trigger/1 -> Subsystem1/Trigger, Subsystem/Trigger, 采样时触发积分并清零/2, MATLAB Function1/1(Trigger)  "Tr"
  延长一个采样时间/1 -> Sum/2, Scope2/1  "上一个采样时刻的Theta"
  Clock/1 -> Subsystem1/1(Timer)
  Sum/1 -> MATLAB Function/1(Theta_error)  "a"
  Subsystem1/1(T_error) -> Scope3/1, 偏差时间/1, MATLAB Function/2(T_error), Gain/1  "计算两个采样冲击之间的时间差"
  Gain/1 -> 延长一个采样时间/2
  MATLAB Function/1(we) -> we/1, Saturation/1
  Memory1/1 -> MATLAB Function/3(a_before)
  采样时触发积分并清零/1 -> Sum1/2
  Sum1/1 -> Scope1/1, Int we/1
  MATLAB Function1/1(y) -> Discrete-Time Integrator/2, Product/1
  Constant/1 -> Product/2
  Product/1 -> Discrete-Time Integrator/1
  Discrete-Time Integrator/1 -> Sum1/1, Scope/1  "补偿第一次积分"
  Saturation/1 -> 采样时触发积分并清零/1, Memory1/1, Scope1/2

== system PIcomper/霍尔传感器/Trigger/Subsystem1 ==
  H1 : Inport
  Detect Decrease : simulink/Logic and Bit Operations/Detect Decrease  vinit=0.0  OutDataTypeStr=boolean
  Detect Increase : simulink/Logic and Bit Operations/Detect Increase  vinit=0.0  OutDataTypeStr=boolean
  OR : Logic  Operator=OR  IconShape=distinctive  AllPortsSameDT=off  OutDataTypeStr=boolean
  Subsystem : Subsystem
  Trigger1 : Outport
  wires:
  Subsystem/1(P1) -> Detect Decrease/1, Detect Increase/1
  H1/1 -> Subsystem/1(Hall-1), Subsystem/Trigger
  Detect Increase/1 -> OR/1
  Detect Decrease/1 -> OR/2
  OR/1 -> Trigger1/1

== system PIcomper/霍尔传感器/Trigger/Subsystem2 ==
  H1 : Inport
  Detect Decrease : simulink/Logic and Bit Operations/Detect Decrease  vinit=0.0  OutDataTypeStr=boolean
  Detect Increase : simulink/Logic and Bit Operations/Detect Increase  vinit=0.0  OutDataTypeStr=boolean
  OR : Logic  Operator=OR  IconShape=distinctive  AllPortsSameDT=off  OutDataTypeStr=boolean
  Subsystem : Subsystem
  Trigger2 : Outport
  wires:
  H1/1 -> Subsystem/1(Hall-1), Subsystem/Trigger
  OR/1 -> Trigger2/1
  Detect Increase/1 -> OR/1
  Detect Decrease/1 -> OR/2
  Subsystem/1(P1) -> Detect Decrease/1, Detect Increase/1

== system PIcomper/霍尔传感器/Trigger/Subsystem3 ==
  note: Trigger2
  H1 : Inport
  Detect Decrease : simulink/Logic and Bit Operations/Detect Decrease  vinit=0.0  OutDataTypeStr=boolean
  Detect Increase : simulink/Logic and Bit Operations/Detect Increase  vinit=0.0  OutDataTypeStr=boolean
  OR : Logic  Operator=OR  IconShape=distinctive  AllPortsSameDT=off  OutDataTypeStr=boolean
  Subsystem : Subsystem
  Trigger3 : Outport
  wires:
  H1/1 -> Subsystem/1(Hall-1), Subsystem/Trigger
  OR/1 -> Trigger3/1
  Detect Increase/1 -> OR/1
  Detect Decrease/1 -> OR/2
  Subsystem/1(P1) -> Detect Decrease/1, Detect Increase/1

== system PIcomper/霍尔传感器/Theta插值处理/计算Hall-Theta之间的加速度——实际上约等于角速度we/Subsystem ==
  Hall-Theta : Inport
  任意沿触发采样 : TriggerPort  TriggerType=either  VariantControl=Variant  PortDimensions=1
  Theta_new : Outport
  wires:
  Hall-Theta/1 -> Theta_new/1

== system PIcomper/霍尔传感器/Theta插值处理/计算Hall-Theta之间的加速度——实际上约等于角速度we/Subsystem1 ==
  Timer : Inport
  任意沿触发采样 : TriggerPort  TriggerType=either  VariantControl=Variant  ShowOutputPort=on  PortDimensions=1
  Delay : Delay
  Scope : Scope  NumInputPorts=3
  Subsystem : Subsystem
  Sum : Sum  Inputs=|+-
  T_error : Outport
  wires:
  Subsystem/1(T1) -> Scope/1, Sum/1, Delay/1
  任意沿触发采样/1 -> Subsystem/Trigger
  Sum/1 -> Scope/2, T_error/1
  Delay/1 -> Sum/2, Scope/3  "T0"
  Timer/1 -> Subsystem/1(Timer)

== system PIcomper/霍尔传感器/Trigger/Subsystem1/Subsystem ==
  Hall-1 : Inport
  任意沿触发采样 : TriggerPort  TriggerType=either  VariantControl=Variant  ShowOutputPort=on  InitialTriggerSignalState=zero  PortDimensions=1
  P1 : Outport
  wires:
  Hall-1/1 -> P1/1

== system PIcomper/霍尔传感器/Trigger/Subsystem2/Subsystem ==
  Hall-1 : Inport
  任意沿触发采样 : TriggerPort  TriggerType=either  VariantControl=Variant  ShowOutputPort=on  InitialTriggerSignalState=zero  PortDimensions=1
  Scope : Scope
  P1 : Outport
  wires:
  任意沿触发采样/1 -> Scope/1
  Hall-1/1 -> P1/1

== system PIcomper/霍尔传感器/Trigger/Subsystem3/Subsystem ==
  Hall-1 : Inport
  任意沿触发采样 : TriggerPort  TriggerType=either  VariantControl=Variant  ShowOutputPort=on  InitialTriggerSignalState=zero  PortDimensions=1
  Scope : Scope
  P1 : Outport
  wires:
  任意沿触发采样/1 -> Scope/1
  Hall-1/1 -> P1/1

== system PIcomper/霍尔传感器/Theta插值处理/计算Hall-Theta之间的加速度——实际上约等于角速度we/Subsystem1/Subsystem ==
  Timer : Inport
  任意沿触发采样 : TriggerPort  TriggerType=either  VariantControl=Variant  PortDimensions=1
  T1 : Outport
  wires:
  Timer/1 -> T1/1

== matlab function PIcomper/BLDC_System/MATLAB Function ==
  data: we input; Hall output; Theta input; psi_f input
function Hall = Hall_sensor(we,Theta,psi_f)

if Theta>=0 && Theta < pi/3
    Hall = [psi_f*we,psi_f*we*((Theta)/(pi/6)-1),-psi_f*we,1,0,0];
elseif Theta>=pi/3 && Theta < 2*pi/3
    Hall = [psi_f*we*((pi/3-Theta)/(pi/6)+1),psi_f*we,-psi_f*we,1,1,0];
elseif Theta>=2*pi/3 && Theta < pi
    Hall = [-psi_f*we,psi_f*we,psi_f*we*((Theta-2*pi/3)/(pi/6)-1),0,1,0];
elseif Theta>=pi && Theta < 4*pi/3
    Hall = [-psi_f*we,psi_f*we*((pi-Theta)/(pi/6)+1),psi_f*we,0,1,1];
elseif Theta>=4*pi/3 && Theta < 5*pi/3
    Hall = [psi_f*we*((Theta-4*pi/3)/(pi/6)-1),-psi_f*we,psi_f*we,0,0,1];
else % Theta>=5*pi/3 && Theta <= 2*pi
    Hall = [psi_f*we,-psi_f*we,psi_f*we*((5*pi/3-Theta)/(pi/6)+1),1,0,1];
end

%% 
% 这里规定
% 100   0~60°-
% 110   60~120°-
% 010   120~180°-
% 011   180~240°-
% 001   240~300°-
% 101   300~360°-

== matlab function PIcomper/霍尔传感器/Theta插值处理/TriggerCounter ==
  data: Trigger input; Counter output
function Counter = fcn(Trigger)
persistent counter
if isempty(counter)
    counter = 0;
end
if Trigger ~= 0
    counter = counter + 1;
else
end

if counter > 6
    counter = 1;
end

Counter = counter;

== matlab function PIcomper/霍尔传感器/Theta插值处理/处理使得每次叠加后角度不超过霍尔基础角度 ==
  data: Hall_Loc input; Theta output; Theta_Hall_Cal input; Theta_Hall input
function Theta = fcn(Hall_Loc, Theta_Hall_Cal, Theta_Hall)
% Theta_hall_Cal 为带有积分的补偿量
% Theta_Hall 为霍尔传感器感应角度
% Counter 为计数器
% 
if Hall_Loc ~= 6
    if Theta_Hall_Cal >= (pi/3)*Hall_Loc
        Theta = (pi/3)*Hall_Loc;
    else
        Theta = Theta_Hall_Cal;
    end
else
    Theta = Theta_Hall_Cal;
end

% if Theta_Hall_Cal >

== matlab function PIcomper/霍尔传感器/Theta插值处理/计算Hall-Theta之间的加速度——实际上约等于角速度we/MATLAB Function ==
  data: Theta_error input; we output; T_error input; a_before input
function we = fcn(Theta_error,T_error,a_before)
persistent Theta_e_p
if isempty(Theta_e_p)
    Theta_e_p = 0;
end

if Theta_error ~= 0
    Theta_e_p = Theta_error;
else
end

if T_error == 0
    we = 0;
elseif Theta_e_p < -pi
    we = a_before;   % 延续上一时刻的加速度
else
    we = Theta_e_p/T_error;
end

== matlab function PIcomper/霍尔传感器/Theta插值处理/计算Hall-Theta之间的加速度——实际上约等于角速度we/MATLAB Function1 ==
  data: Trigger input; y output
function y = fcn(Trigger)
persistent k
if isempty(k)
    k = 0;
end

if Trigger ~= 0
    k = k + 1; % 记录触发次数k
end

% 仅在第一次触发时，添加积分
if k == 1
    y = 40;
else
    y = 0;
end

== matlab function PIcomper/霍尔传感器/计算Theta角度/MATLAB Function ==
  data: Hall_abc input; theta_Hall output; theta_loc output
function [theta_Hall,theta_loc]= Cal_Theta(Hall_abc)

% 转一个二进制对应（注意这里是从左往右，实际上为了对应简单而已）
Number = Hall_abc(1)*1 + Hall_abc(2)*2 + Hall_abc(3)*4;

if Number == 1
    theta_Hall = 0;
    theta_loc = 1;
elseif Number == 3
    theta_Hall = pi/3;
    theta_loc = 2;
elseif Number == 2
    theta_Hall = 2*pi/3;
    theta_loc = 3;
elseif Number == 6
    theta_Hall = pi;
    theta_loc = 4;
elseif Number == 4
    theta_Hall = 4*pi/3;
    theta_loc = 5;
else    % elseif Hall_abc == 101
    theta_Hall = 5*pi/3;
    theta_loc = 6;
end

%% 前面规定
%   1   100   0~60°-
%   3   110   60~120°-
%   2   010   120~180°-
%   6   011   180~240°-
%   4   001   240~300°-
%   5   101   300~360°-

== matlab function PIcomper/参考电流/当前位置+参考电流生成三相参考电流 ==
  settings: updateMethod=DISCRETE
  data: I_ref input; Iabc_Ref output size=[1 3]; theta input
function Iabc_Ref = fcn(I_ref,theta)
% persistent Iabc_ref;
% if isempty(Iabc_ref)
%     Iabc_ref = [0, 0, 0];
% end

if theta>=0 && theta <= pi/3
    Iabc_ref = [I_ref,0,-I_ref];
elseif theta>=pi/3 && theta <= 2*pi/3
    Iabc_ref = [0,I_ref,-I_ref];
elseif theta>=2*pi/3 && theta <= pi
    Iabc_ref = [-I_ref,I_ref,0];
elseif theta>=pi && theta <= 4*pi/3
    Iabc_ref = [-I_ref,0,I_ref];
elseif theta>=4*pi/3 && theta <= 5*pi/3
    Iabc_ref = [0,-I_ref,I_ref];
else % theta>=5*pi/3 && theta <= 2*pi
    Iabc_ref = [I_ref,-I_ref,0];
end

Iabc_Ref = Iabc_ref;
